simulink model "rtctrl"  (Simulink 6.0)
settings: Solver=ode4  StartTime=0.0  StopTime=10.0  RelTol=1e-3
libraries: rtwinlib x2, simulink_extras x1
settings Model: Creator=Houska  LastModifiedBy=Houska  ExtModeMexFile=rtwinext  ExtModeTrigDuration=10000  ProdHWDeviceType=32-bit Real-Time Windows Target
settings ConfigSet: SimulationMode=external
settings DataIOCC: SaveOutput=off  SaveTime=off  SignalLoggingName=logsOut
settings OptimizationCC: MultiInstanced=off
settings FormatCC: IgnoreBidirectionalLines=off
settings HardwareCC: ProdIntDivRoundTo=Zero  ProdEndianess=LittleEndian  ProdHWDeviceType=32-bit Real-Time Windows Target
settings RTWCC: SystemTargetFile=rtwin.tlc  TemplateMakefile=rtwin.tmf  Description=Real-Time Windows Target  ProcessScript=rtwin_make_rtw_hook
settings CodeAppCC: SimulinkBlockComments=off
settings RTWinTargetCC: TargetFcnLib=iso_c_tmw.mat  CCOptimize=on

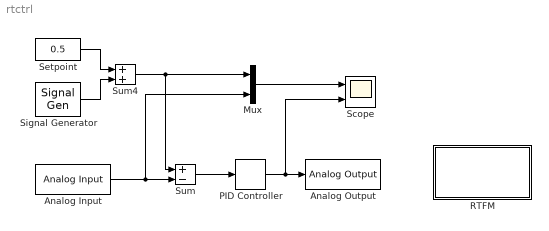
== system rtctrl ==
  Analog Input : rtwinlib/Analog Input  SampleTime=1e-3  DrvAddress=0  DrvOptions=0  Channels=1  RangeMode=1  VoltRange=1
  Analog Output : rtwinlib/Analog Output  SampleTime=1e-3  DrvAddress=0  DrvOptions=0  Channels=1  RangeMode=1  VoltRange=1  InitialValue=[]  FinalValue=[]
  Mux : Mux  Inputs=2
  PID Controller : simulink_extras/Additional Linear/PID Controller  P=4  I=40  D=0.08
  "RTFM " : Subsystem
      mask Type: Frame-Based Simulation Info
      mask Display: disp('Info')
  Scope : Scope  NumInputPorts=2
      settings: TimeRange=10  YMin=-5~-5  YMax=5~5  DataFormat=Structure
  Setpoint : Constant  Value=0.5
  Signal Generator : SignalGenerator  WaveForm=square  Amplitude=0.20000  Frequency=3.000000  Units=rad/sec
  Sum : Sum  Inputs=+-  SaturateOnIntegerOverflow=on  InputSameDT=on
  Sum4 : Sum  SaturateOnIntegerOverflow=on  InputSameDT=on
  wires:
  Setpoint/1 -> Sum4/1
  Signal Generator/1 -> Sum4/2
  Sum4/1 -> Sum/1, Mux/1
  Analog Input/1 -> Sum/2, Mux/2
  PID Controller/1 -> Analog Output/1, Scope/2
  Sum/1 -> PID Controller/1
  Mux/1 -> Scope/1

== system rtctrl/RTFM  ==
  note: How to run this demo:
      |
      | 1) Open the Analog Input and Analog Output blocks and select your
      |     data acquisition board.
      |     If there's no board installed, install it using the Install new board button.
      | 2) Build the model using Tools->Real-Time Workshop->Build Model.
      | 3) Connect to the real-time code using Simulation->Connect to target.
      | 4) Start the real-time execution using Simulation->Start real-time code.
      |
      | Note: To run this demo, you must have a data acquisition board plugged into
      | your computer.
